simulink model "buck_boost_regulacija_fin"  (R2025a)
settings: Solver=FixedStepAuto  StartTime=0.0  StopTime=3  FixedStep=0.001  RelTol=1e-3
values from neighbouring files (symbols this model uses):
  C = 470e-6    (= 0.00047)    [projekat_1.m]
  den_NF_INV = [1/300 1]    [projekat_1.m]
  den_NF_PI = [1/50 1]    [projekat_1.m]
  den_NF_ZN = [1/400 1]    [projekat_1.m]
  E = 12    [projekat_1.m]
  L = 15.91e-3    (= 0.01591)    [projekat_1.m]
  noise_var = (0.03*x2_eq)^2    (= 0.455625)    [projekat_1.m]
  num_NF_INV = [1]    [projekat_1.m]
  num_NF_PI = [1]    [projekat_1.m]
  num_NF_ZN = [1]    [projekat_1.m]
  R = 52    [projekat_1.m]
  sel = sels(i)    [projekat_1.m]
  u_eq = eval(u_eq)    [projekat_1.m]
  x2_eq = -22.5    [projekat_1.m]
undefined symbols (not defined in the file or in its folder): den1, den2, den_INV, den_PI, num1, num2, num_INV, num_PI
settings Model: Creator=PC  LastModifiedBy=PC
settings DataIOCC: ReturnWorkspaceOutputs=off

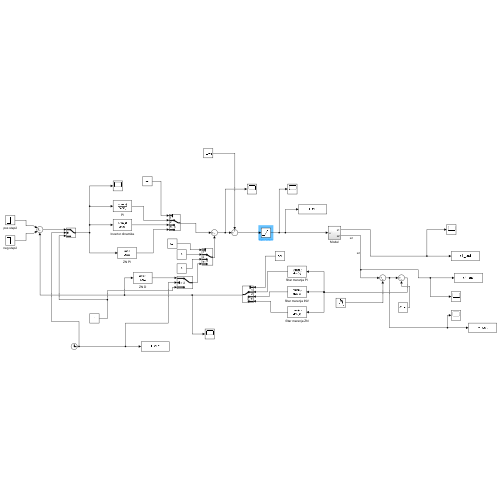
[thumbnail: Simulink's stored preview of the top-level diagram]
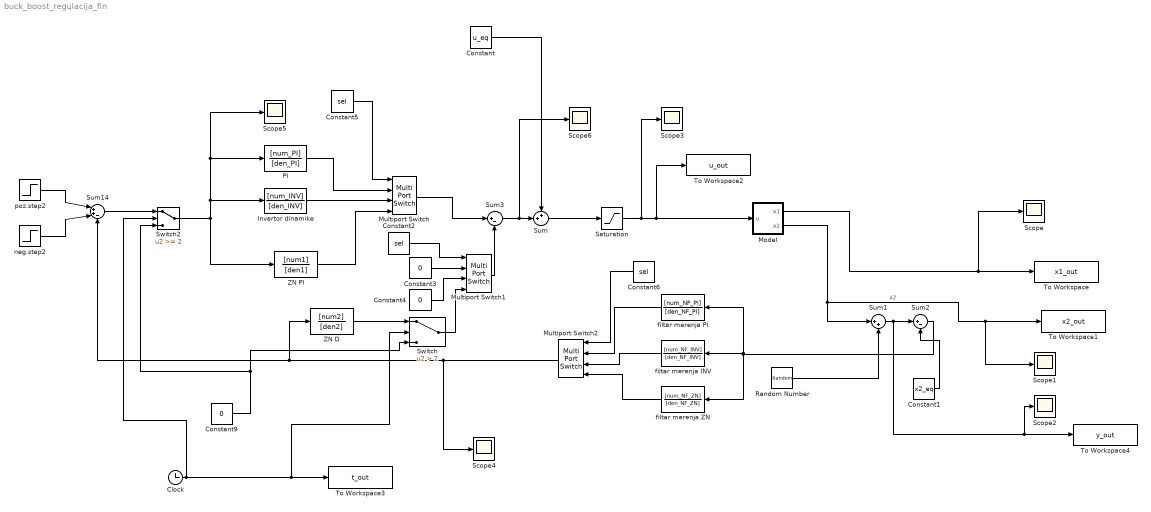
== system buck_boost_regulacija_fin ==
  Clock : Clock
  Constant : Constant  Value=u_eq
  Constant1 : Constant  Value=x2_eq
  Constant2 : Constant  Value=sel
  Constant3 : Constant  Value=0
  Constant4 : Constant  Value=0
  Constant5 : Constant  Value=sel
  Constant6 : Constant  Value=sel
  Constant9 : Constant  Value=0
  Invertor dinamike : TransferFcn  Numerator=[num_INV]  Denominator=[den_INV]
  Model : Subsystem
  Multiport Switch : MultiPortSwitch  SaturateOnIntegerOverflow=off  InputSameDT=off
  Multiport Switch1 : MultiPortSwitch  SaturateOnIntegerOverflow=off  InputSameDT=off
  Multiport Switch2 : MultiPortSwitch  SaturateOnIntegerOverflow=off  InputSameDT=off
  PI : TransferFcn  Numerator=[num_PI]  Denominator=[den_PI]
  Random Number : RandomNumber  Variance=noise_var  SampleTime=0.001
  Saturation : Saturate  UpperLimit=0.90  LowerLimit=0.20
  Scope{,1..6} (7 alike) : Scope
      Scope settings: ActiveDisplayYMinimum=-1  ActiveDisplayYMaximum=1
      Scope1 settings: ActiveDisplayYMinimum=-17.390570872112225  ActiveDisplayYMaximum=17.699619428483988
      Scope2 settings: ActiveDisplayYMinimum=-1.226762900906336E+223  ActiveDisplayYMaximum=1.0997258244058199E+223  DataLoggingVariableName=ScopeData2
      Scope3 settings: ActiveDisplayYMinimum=0.32966598731056374  ActiveDisplayYMaximum=1.018752292305293  DataLoggingVariableName=ScopeData3
      Scope4 settings: ActiveDisplayYMinimum=-20.327822254462426  ActiveDisplayYMaximum=5.8570180187516909  DataLoggingVariableName=ScopeData4
      Scope5 settings: ActiveDisplayYMinimum=-0.83588221436992782  ActiveDisplayYMaximum=30.064451899251992  DataLoggingVariableName=ScopeData5
      Scope6 settings: ActiveDisplayYMinimum=-132.7226298777324  ActiveDisplayYMaximum=31.716936684348454  DataLoggingVariableName=ScopeData6
  Sum : Sum  Inputs=++|
  Sum1 : Sum  Inputs=|++
  Sum14 : Sum  Inputs=|++-
  Sum2 : Sum  Inputs=|+-
  Sum3 : Sum  Inputs=|+-
  Switch : Switch  Criteria=u2 > Threshold  Threshold=2  SaturateOnIntegerOverflow=off  InputSameDT=off
  Switch2 : Switch  Threshold=2  SaturateOnIntegerOverflow=off  InputSameDT=off
  To Workspace : ToWorkspace  VariableName=x1_out  SampleTime=-1
  To Workspace1 : ToWorkspace  VariableName=x2_out  SampleTime=-1
  To Workspace2 : ToWorkspace  VariableName=u_out  SampleTime=-1
  To Workspace3 : ToWorkspace  VariableName=t_out  SampleTime=-1
  To Workspace4 : ToWorkspace  VariableName=y_out  SampleTime=-1
  ZN D : TransferFcn  Numerator=[num2]  Denominator=[den2]
  ZN PI : TransferFcn  Numerator=[num1]  Denominator=[den1]
  filtar merenja INV : TransferFcn  Numerator=[num_NF_INV]  Denominator=[den_NF_INV]
  filtar merenja PI : TransferFcn  Numerator=[num_NF_PI]  Denominator=[den_NF_PI]
  filtar merenja ZN : TransferFcn  Numerator=[num_NF_ZN]  Denominator=[den_NF_ZN]
  neg.step2 : Step  Time=3  After=-5  SampleTime=0
  poz.step2 : Step  Time=2  After=5  SampleTime=0
  wires:
  Saturation/1 -> Scope3/1, To Workspace2/1, Model/1(u)
  Model/1(x1) -> Scope/1, To Workspace/1
  Sum1/1 -> To Workspace4/1, Scope2/1, Sum2/1
  Random Number/1 -> Sum1/2
  Sum/1 -> Saturation/1
  Constant/1 -> Sum/1
  Constant9/1 -> Switch2/3, Switch/3
  neg.step2/1 -> Sum14/2
  Sum14/1 -> Switch2/1
  poz.step2/1 -> Sum14/1
  Model/2(x2) -> Sum1/1, Scope1/1, To Workspace1/1  "x2"
  Constant1/1 -> Sum2/2
  Clock/1 -> Switch/2, To Workspace3/1, Switch2/2
  Sum2/1 -> filtar merenja PI/1, filtar merenja INV/1, filtar merenja ZN/1
  Sum3/1 -> Scope6/1, Sum/2
  ZN D/1 -> Switch/1
  filtar merenja ZN/1 -> Multiport Switch2/4
  Multiport Switch/1 -> Sum3/1
  ZN PI/1 -> Multiport Switch/4
  Multiport Switch1/1 -> Sum3/2
  Switch/1 -> Multiport Switch1/4
  Constant2/1 -> Multiport Switch1/1
  Constant3/1 -> Multiport Switch1/2
  Constant4/1 -> Multiport Switch1/3
  Constant5/1 -> Multiport Switch/1
  Switch2/1 -> Invertor dinamike/1, Scope5/1, PI/1, ZN PI/1
  PI/1 -> Multiport Switch/2
  Invertor dinamike/1 -> Multiport Switch/3
  Multiport Switch2/1 -> Scope4/1, Sum14/3, ZN D/1
  Constant6/1 -> Multiport Switch2/1
  filtar merenja INV/1 -> Multiport Switch2/3
  filtar merenja PI/1 -> Multiport Switch2/2

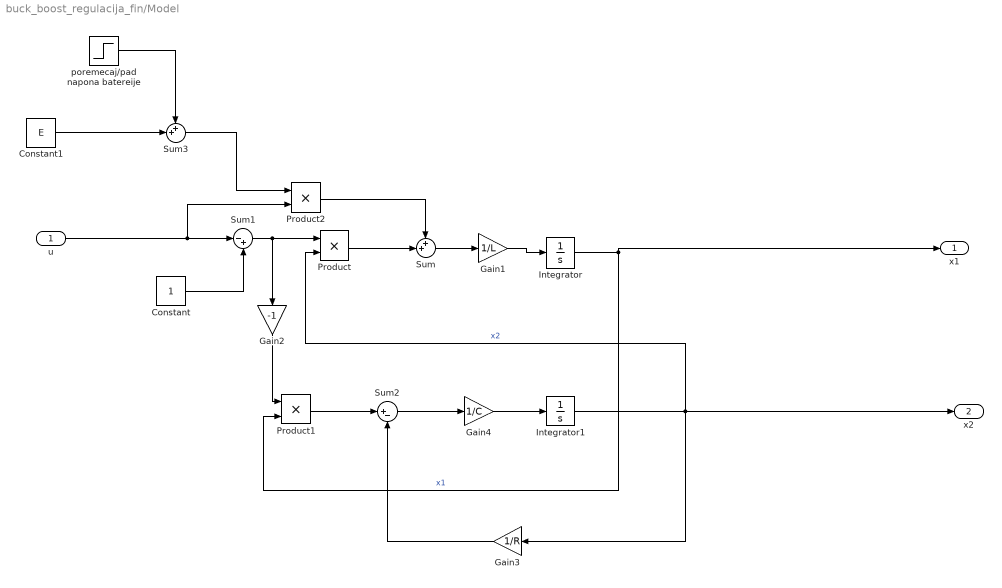
== system buck_boost_regulacija_fin/Model ==
  u : Inport
  Constant : Constant
  Constant1 : Constant  Value=E
  Gain1 : Gain  Gain=1/L
  Gain2 : Gain  Gain=-1
  Gain3 : Gain  Gain=1/R
  Gain4 : Gain  Gain=1/C
  Integrator : Integrator  LimitOutput=on  LowerSaturationLimit=0
  Integrator1 : Integrator  LimitOutput=on  UpperSaturationLimit=0
  Product : Product
  Product1 : Product
  Product2 : Product
  Sum : Sum  Inputs=++|
  Sum1 : Sum  Inputs=|-+
  Sum2 : Sum  Inputs=|+-
  Sum3 : Sum  Inputs=++|
  poremecaj/pad napona batereije : Step  Time=4.5  After=-1  SampleTime=0
  x1 : Outport
  x2 : Outport  Port=2
  wires:
  Product1/1 -> Sum2/1
  Integrator1/1 -> x2/1, Gain3/1, Product/2  "x2"
  Gain3/1 -> Sum2/2
  Constant/1 -> Sum1/2
  Sum2/1 -> Gain4/1
  Product/1 -> Sum/2
  Gain1/1 -> Integrator/1
  Sum1/1 -> Product/1, Gain2/1
  Integrator/1 -> x1/1, Product1/2  "x1"
  Product2/1 -> Sum/1
  u/1 -> Product2/2, Sum1/1
  Gain4/1 -> Integrator1/1
  Sum/1 -> Gain1/1
  Gain2/1 -> Product1/1
  Constant1/1 -> Sum3/2
  poremecaj/pad napona batereije/1 -> Sum3/1
  Sum3/1 -> Product2/1
